simulink model "predatpr_prey"  (R2021b)
settings: Solver=ode45  StartTime=0.0  StopTime=1000  MaxStep=0.001  RelTol=1e-3
undefined symbols (not defined in the file or in its folder): bx, rx
settings Model: Creator=francesco  LastModifiedBy=francesco

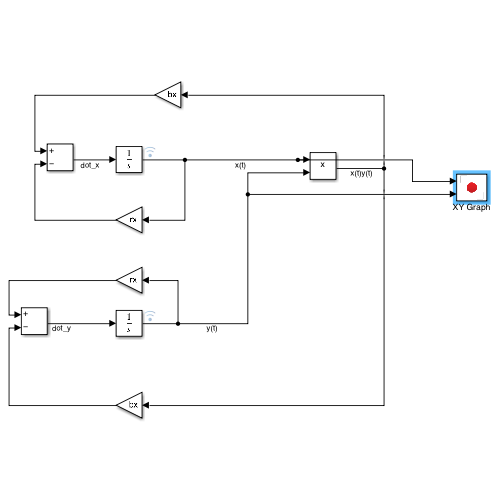
[thumbnail: Simulink's stored preview of the top-level diagram]
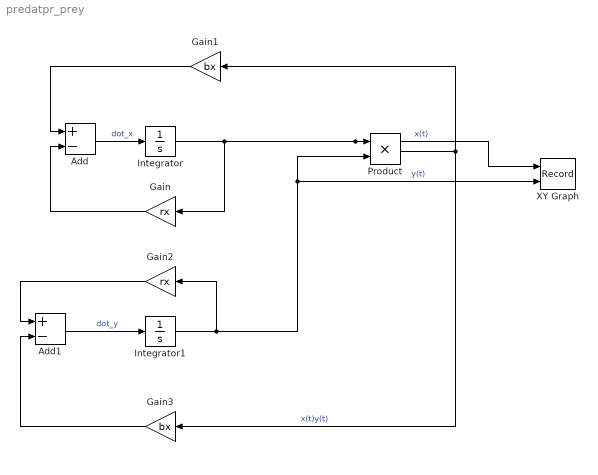
== system predatpr_prey ==
  Add : Sum  Inputs=+-
  Add1 : Sum  Inputs=+-
  Gain : Gain  Gain=rx
  Gain1 : Gain  Gain=bx
  Gain2 : Gain  Gain=rx
  Gain3 : Gain  Gain=bx
  Integrator : Integrator  InitialCondition=1
  Integrator1 : Integrator  InitialCondition=3
  Product : Product
  XY Graph : Record  FileSettingsInternal="{\"entries\":[{\"content\":{\"excelSettings\":{\"content\":{},\"type\":\"Streamout.ExcelSettings\"}},\"type\":\"Streamout.FileSettingStorage\",\"uuid\":\"3d654736-06dc-4bd4-becb-4502d05f82b1\"}],\"packageUris\":[\"http://schema.mathworks.com/mf0/streamout_blocks/R2020a\"],\"version\":\"1.0\"}"  Layout=[1 1]  SignalsInternal="{\"entries\":[{\"content\":{\"signals\":[{\"content\":{\"blockPath\":[\"untitled/XY Graph\"],\"channel\":[],\"dimensions\":[1],\"domain\":\"untitled/XY Graph\",\"lineColor\":\"#a2142f\",\"plots\":[1],\"port\":1,\"sid\":[\"\"],\"signalID\":335,\"signalName\":\"x(t)\"},\"type\":\"RecordBlkView.Signal\",\"uuid\":\"934532f6-ad64-45ec-80f3-9f0814c1c69c\"},{\"content\":{\"blockPath\":[\"untitled/XY Graph\"],\"channel\":[],\"dimensions\":[1],\"domain\":\"untitled/XY Graph\",\"lineColor\":\"#139fff\",\"plots\":[1],\"port\":2,\"sid\":[\"\"],\"signalID\":339,\"signalName\":\"y(t)\"},\"type\":\"RecordBlkView.Signal\",\"uuid\":\"868dcba4-05d7-49ea-8527-00d2bf700dfb\"}]},\"type\":\"RecordBlkView.InputSignals\",\"uuid\":\"e3c09483-d315-40b1-a172-3198e972b399\"}],\"packageUris\":[\"http://schema.mathworks.com/mf0/streamout_blocks/R2020a\"],\"version\":\"1.0\"}"  VisualizationBindings="{\"xyplotplugin\":{\"info\":[{\"series\":[{\"bindingParametersList\":[{\"parameter\":\"X-Axis\",\"signalID\":335,\"signalName\":\"x(t)\"},{\"parameter\":\"Y-Axis\",\"signalID\":339,\"signalName\":\"y(t)\"}],\"seriesID\":63553}],\"subplotID\":1}]}}"  CompatibilityTag=XY
  wires:
  Add/1 -> Integrator/1  "dot_x"
  Integrator/1 -> Gain/1, XY Graph/1, Product/1  "x(t)"
  Gain/1 -> Add/2
  Product/1 -> Gain1/1, Gain3/1  "x(t)y(t)"
  Gain1/1 -> Add/1
  Add1/1 -> Integrator1/1  "dot_y"
  Integrator1/1 -> Gain2/1, XY Graph/2, Product/2  "y(t)"
  Gain2/1 -> Add1/1
  Gain3/1 -> Add1/2
